simulink model "inner_hair_cell"  (R2020b)
settings: Solver=FixedStepDiscrete  StartTime=0.0  StopTime=stopTime  FixedStep=2.0833333333333333e-05  RelTol=1e-3
undefined symbols (not defined in the file): ihcasym_c1, ihcasym_c2, mp, slope_c1, slope_c2
settings Model: Creator=Ross  LastModifiedBy=conno
settings DataIOCC: SaveOutput=off  SaveTime=off  ReturnWorkspaceOutputs=off
settings OptimizationCC: BlockReduction=off  ConditionallyExecuteInputs=off  DefaultParameterBehavior=Inlined
settings DebuggingCC: ReadBeforeWriteMsg=DisableAll  WriteAfterWriteMsg=DisableAll  WriteAfterReadMsg=DisableAll  AlgebraicLoopMsg=error  MultiTaskDSMMsg=none  SingleTaskRateTransMsg=error  PregeneratedLibrarySubsystemCodeDiagnostic=none  ArithmeticOperatorsInVariantConditions=warning
settings HardwareCC: ProdBitPerPointer=32  ProdBitPerSizeT=32  ProdBitPerPtrDiffT=32  ProdLargestAtomicFloat=None  ProdIntDivRoundTo=Undefined  ProdEndianess=Unspecified  ProdWordSize=32  ProdHWDeviceType=ASIC/FPGA->ASIC/FPGA  TargetBitPerPointer=64  TargetBitPerSizeT=64  TargetBitPerPtrDiffT=64  TargetLongLongMode=on  TargetIntDivRoundTo=Zero  TargetEndianess=LittleEndian  TargetWordSize=64  TargetHWDeviceType=Custom Processor->MATLAB Host Computer  ProdEqTarget=off
settings ModelReferenceCC: UpdateModelReferenceTargets=IfOutOfDate
settings SFSimCC: SFSimEcho=off  SimUseLocalCustomCode=off  CustomCodeUndefinedFunction=UseInterfaceOnly
settings RTWCC: RTWUseLocalCustomCode=off

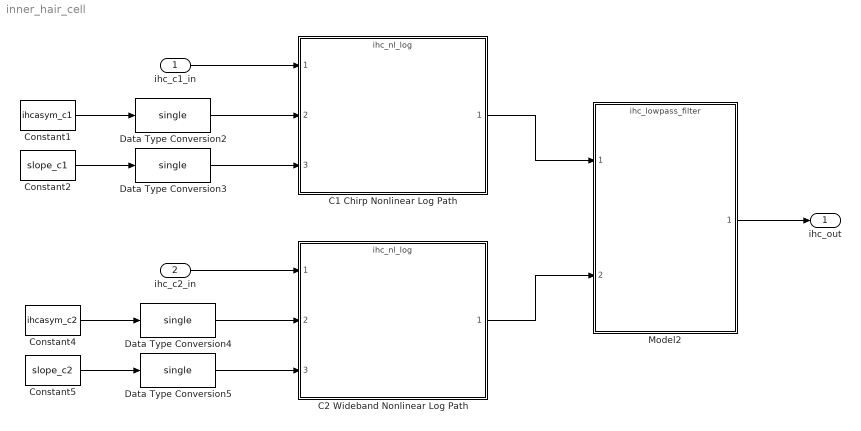
== system inner_hair_cell ==
  ihc_c1_in : Inport  OutDataTypeStr=single  PortDimensions=1  SampleTime=[2.0833333333333333e-05,0]
  ihc_c2_in : Inport  Port=2  OutDataTypeStr=single  PortDimensions=1  SampleTime=[2.0833333333333333e-05,0]
  C1 Chirp Nonlinear Log Path : ModelReference  ModelNameDialog=ihc_nl_log.slx  SimulationMode=Normal  ModelReferenceVersion=1.125
  C2 Wideband Nonlinear Log Path : ModelReference  ModelNameDialog=ihc_nl_log.slx  SimulationMode=Normal  ModelReferenceVersion=1.125
  Constant1 : Constant  Value=ihcasym_c1  SampleTime=mp.Ts_sim
  Constant2 : Constant  Value=slope_c1  SampleTime=mp.Ts_sim
  Constant4 : Constant  Value=ihcasym_c2  SampleTime=mp.Ts_sim
  Constant5 : Constant  Value=slope_c2  SampleTime=mp.Ts_sim
  Data Type Conversion{2..5} (4 alike) : DataTypeConversion  OutDataTypeStr=single
  Model2 : ModelReference  ModelNameDialog=ihc_lowpass_filter.slx  SimulationMode=Normal  ModelReferenceVersion=1.124
  ihc_out : Outport  OutDataTypeStr=single  PortDimensions=1  SampleTime=[2.0833333333333333e-05,0]  InitialOutput=0  VectorParamsAs1DForOutWhenUnconnected=off
  wires:
  C1 Chirp Nonlinear Log Path/1 -> Model2/1
  Model2/1 -> ihc_out/1
  ihc_c1_in/1 -> C1 Chirp Nonlinear Log Path/1
  ihc_c2_in/1 -> C2 Wideband Nonlinear Log Path/1
  C2 Wideband Nonlinear Log Path/1 -> Model2/2
  Data Type Conversion2/1 -> C1 Chirp Nonlinear Log Path/2
  Constant2/1 -> Data Type Conversion3/1
  Constant1/1 -> Data Type Conversion2/1
  Constant4/1 -> Data Type Conversion4/1
  Constant5/1 -> Data Type Conversion5/1
  Data Type Conversion4/1 -> C2 Wideband Nonlinear Log Path/2
  Data Type Conversion5/1 -> C2 Wideband Nonlinear Log Path/3
  Data Type Conversion3/1 -> C1 Chirp Nonlinear Log Path/3
